simulink model "TRN_V3_2"  (R2022a)
settings: Solver=FixedStepAuto  StartTime=0.0  StopTime=300  FixedStep=0.04  RelTol=1e-3
PreLoadFcn:
  | load('BusStructureTRNsensor.mat');
  | addpath('C:/MAP');
InitFcn:
  | %load TRNDataBusPILS.mat
  | %addpath(genpath(cd))
  | 
  | %load('TPF_WHOLESIM_INPUT_SCENARIOS_AGCAS_N35_10E127_70.mat');
  | 
  | % Add DataBus Path
  | addpath(',,/');
  | addpath('../MAP/');
  | addpath('../MAP/MAP_DB');
  | addpath('../MAP/DVOF');
  | addpath(genpath(cd));
  | load('BusStructureTRN.mat');
undefined symbols (not defined in the file or in its folder): Altitude_INS, Latitude_INS, Longitude_INS, residual, Result_Prev, TimeTag_Prev, TRN, TRNlib
libraries: simulink_extras x21, sharedtransform x2
(part 4 of 4)

== stateflow chart TRN_V3_2/TRN/ModeManagementCSU ==
  state Operation_In_Flight
    state Terrain_Referenced_Navigation [parallel]
      settings: executionOrder=1
      state TrackingCSU
        state ContinuousUpdate [parallel]
          en,du:
          [latINSErrTRN, lonINSErrTRN, altINSErrTRN, Out_TRNOutput.TRNHorUncertainty, ...
          Out_TRNOutput.TRNVerticalUncertainty, Out_TRNDatapump] = TrackingCSU(In_TRNInput,Qmatrix, In_TRNDatapump);
          [continuousValid, Out_TRNOutput.NavigationMode]...
          = CheckValidity( Out_TRNOutput.TRNHorUncertainty, In_TRNInput.INSDataNotValid, In_TRNInput.INS_Alignment_State, ...
          In_TRNInput.GPSDataNotValid);
          [Out_TRNOutput.TRN_Ver_FlightPath_Angle] = Ver_FlightPath_Angle(In_TRNInput);
          settings: executionOrder=1
        state ContinuousValid [parallel]
          en, du:
          [Out_TRNOutput.TRNEstOfINSLatitudeErr, Out_TRNOutput.TRNEstOfINSLongitudeErr, Out_TRNOutput.TRNEstOfINSAltitudeErr, ...
          Out_TRNOutput.AircraftPositionCorrectionValid] ...
          = ValidityCheck(continuousValid, latINSErrTRN, lonINSErrTRN, altINSErrTRN, Out_TRNDatapump.Result_Prev);
          settings: executionOrder=2
      state AcquisitionCSU
        state Batch_On
          state StoreProfile [parallel]
            en, du: [Out_TRNDatapump.MAD, Out_TRNDatapump.profileCnt, posUpdate, Out_TRNDatapump.residual(1)] =...
            AcquisitionCSU(In_TRNInput,In_TRNDatapump);
            settings: executionOrder=1
          state BatchUpdate_Valid [parallel]
            en, du:
            [Out_TRNOutput.TRNEstOfINSLatitudeErr, Out_TRNOutput.TRNEstOfINSLongitudeErr, Out_TRNOutput.TRNEstOfINSAltitudeErr, ...
            Out_TRNDatapump.profileCnt, Out_TRNOutput.NavigationMode, Out_TRNOutput.AircraftPositionCorrectionValid ] = ...
            CorrelationValid(Out_TRNDatapump, In_TRNInput, posUpdate);
            [Out_TRNOutput.TRN_Ver_FlightPath_Angle] = Ver_FlightPath_Angle(In_TRNInput);
            settings: executionOrder=2
        state Batch_Idle
          entry: Out_TRNOutput.TRNEstOfINSLatitudeErr = 0.0;
          Out_TRNOutput.TRNEstOfINSLongitudeErr = 0.0;
          Out_TRNOutput.NavigationMode = true;
          Out_TRNOutput.AircraftPositionCorrectionValid = false;
        (default) -> Batch_On
        Batch_Idle -> Batch_On : after(24, tick)
        Batch_On -> Batch_Idle : after(1, tick)
      (default) -> AcquisitionCSU
      TrackingCSU -> AcquisitionCSU : [In_TRNOutput.NavigationMode == true || ...
          | In_TRNInput.SoftResetRequest == true]
      AcquisitionCSU -> TrackingCSU : [In_TRNOutput.NavigationMode == false]
  state Flight_Idle
    en, du:
    [Out_TRNOutput.TRN_Ver_FlightPath_Angle] = Ver_FlightPath_Angle(In_TRNInput);
    Out_TRNOutput.TRN_valid = true;
    Out_TRNOutput.TRNEstOfINSLatitudeErr = 0.0;
    Out_TRNOutput.TRNEstOfINSLongitudeErr = 0.0;
    Out_TRNOutput.TRNEstOfINSAltitudeErr = 0.0;
    Out_TRNOutput.NavigationMode = false;
    Out_TRNOutput.AircraftPositionCorrectionValid = false;
  state [latINSErrTRN, lonINSErrTRN, altINSErrTRN, hUncertainty, vUncertainty, Out_TRNDatapump] ... [function]
    = TrackingCSU(In_TRNInput,Qmatrix,In_TRNDatapump)
  state [MAD,profileCnt,posUpdate,residual] ... [function]
    = AcquisitionCSU(In_TRNInput,In_TRNDatapump)
  state [TRNEstLatErr,TRNEstLonErr,TRNEstAltErr,profileCnt,NavigationMode,AircraftPositionCorrectionValid] = CorrelationValid(In_TRNDatapump,In_TRNInput,posUpdate) [function]
  state [TRNEstOfINSLatitudeErr,TRNEstOfINSLongitudeErr,TRNEstOfINSAltitudeErr,AircraftPositionCorrectionValid] ... [function]
    = ValidityCheck(continuousValid,latINSErrTRN,lonINSErrTRN,altINSErrTRN,Result_prev)
  state TRN_Ver_FlightPath_Angle = Ver_FlightPath_Angle(In_TRNInput) [function]
  (default) -> Operation_In_Flight
  Operation_In_Flight -> Flight_Idle : [In_TRNInput.WeightOnWheels == true]
  Flight_Idle -> Operation_In_Flight : [In_TRNInput.WeightOnWheels == false]
  data: In_TRNInput function_input Bus: TRNInput size=1 =0; Qmatrix function_input double size=[6 6]; latINSErrTRN function_output; lonINSErrTRN function_output; altINSErrTRN function_output; hUncertainty function_output; vUncertainty function_output; In_TRNDatapump function_input Bus: TRNDatapump size=1; Out_TRNDatapump function_output; In_TRNInput function_input Bus: TRNInput size=1 =0; In_TRNDatapump function_input Bus: TRNDatapump size=1 =0; MAD function_output; profileCnt function_output; posUpdate function_output; residual function_output; In_TRNDatapump function_input Bus: TRNDatapump size=1; TRNEstLatErr function_output; TRNEstLonErr function_output; TRNEstAltErr function_output; In_TRNInput function_input Bus: TRNInput size=1; profileCnt function_output uint32; NavigationMode function_output boolean; AircraftPositionCorrectionValid function_output; posUpdate function_input double size=2; hUncertaintyTRN function_input; INSDataNotValid function_input; valid function_output; navigationMode function_output; INS_Alignment_State function_input; GPSDataNotValid function_input; TRNEstOfINSLatitudeErr function_output; TRNEstOfINSLongitudeErr function_output; TRNEstOfINSAltitudeErr function_output; AircraftPositionCorrectionValid function_output boolean; continuousValid function_input boolean size=1; latINSErrTRN function_input double size=1; lonINSErrTRN function_input double size=1; altINSErrTRN function_input double size=1; Result_prev function_input uint16 size=6; In_TRNInput function_input Bus: TRNInput size=1; TRN_Ver_FlightPath_Angle function_output double; In_TRNInput input Bus: TRNInput; In_TRNOutput input Bus: TRNOutput; In_TRNDatapump input Bus: TRNDatapump; Out_TRNOutput output Bus: TRNOutput; Out_TRNDatapump output Bus: TRNDatapump; Qmatrix input double size=[6 6]; lonINSErrTRN local double; latINSErrTRN local double; altINSErrTRN local double; continuousValid local boolean; posUpdate local
  function [valid, navigationMode] = CheckValidity(hUncertaintyTRN, INSDataNotValid, INS_Alignment_State, GPSDataNotValid):
    | function [valid, navigationMode] = CheckValidity(hUncertaintyTRN, INSDataNotValid, INS_Alignment_State, GPSDataNotValid)
    | 
    | persistent invalidCnt
    | if(isempty(invalidCnt))
    |     invalidCnt = 0;
    | end
    | 
    | 
    | if GPSDataNotValid == true
    |     if(hUncertaintyTRN > (256)) || INS_Alignment_State == false
    |         valid = false;
    |         invalidCnt = invalidCnt + 1;
    |     else
    |         valid = true;
    |         invalidCnt = 0;
    |     end
    | else
    |     if(hUncertaintyTRN > 256)
    |         valid = false;
    |         invalidCnt = invalidCnt + 1;
    |     else
    |         valid = true;
    |         invalidCnt = 0;
    |     end
    | end
    | 
    | if GPSDataNotValid == true
    |     if (invalidCnt > 50) || (INSDataNotValid == true)
    |         navigationMode = true;        % Acq CSU
    |     else
    |         navigationMode = false;       % Track CSU
    |     end
    | else
    |     if (invalidCnt > 50)
    |         navigationMode = true;        % Acq CSU
    |     else
    |         navigationMode = false;       % Track CSU
    |     end
    | end
    | if navigationMode == true
    |     invalidCnt = 0;
    | end
    | end

== matlab function TRN_V3_2/TRN/ModeManagementCSU/AcquisitionCSU/AcquisitionCSU/StoreProfile ==
  data: firstRun input; profileCnt output; batchProfile output; gridSize output; latINS input; lonINS input; altINS input; RALT input; latGPS input; lonGPS input; altGPS input; GPSDataNotValid input; flagINS input; GPSFoM input; batchProfile input; profileCnt input; gridSize input; MAPvalidFlag input
function [profileCnt, batchProfile, gridSize] = StoreProfile(firstRun, latINS, lonINS, altINS, RALT, latGPS, lonGPS, altGPS, GPSDataNotValid, flagINS, GPSFoM, batchProfile, profileCnt, gridSize, MAPvalidFlag)

if (GPSDataNotValid == false) && (GPSFoM <= 2)

    batchProfile((profileCnt*(3+((gridSize + gridSize + 1) * (gridSize + gridSize + 1)))) + 1) = altGPS - RALT;
    batchProfile((profileCnt*(3+((gridSize + gridSize + 1) * (gridSize + gridSize + 1)))) + 2) = latGPS;
    batchProfile((profileCnt*(3+((gridSize + gridSize + 1) * (gridSize + gridSize + 1)))) + 3) = lonGPS;
    
    if firstRun == true
        batchProfile((profileCnt*(3+((gridSize + gridSize + 1) * (gridSize + gridSize + 1)))) + 1) = altINS - RALT;
        batchProfile((profileCnt*(3+((gridSize + gridSize + 1) * (gridSize + gridSize + 1)))) + 2) = latINS;
        batchProfile((profileCnt*(3+((gridSize + gridSize + 1) * (gridSize + gridSize + 1)))) + 3) = lonINS;
    end

else
    batchProfile((profileCnt*(3+((gridSize + gridSize + 1) * (gridSize + gridSize + 1)))) + 1) = altINS - RALT;
    batchProfile((profileCnt*(3+((gridSize + gridSize + 1) * (gridSize + gridSize + 1)))) + 2) = latINS;
    batchProfile((profileCnt*(3+((gridSize + gridSize + 1) * (gridSize + gridSize + 1)))) + 3) = lonINS;

end

if (flagINS == false) && (MAPvalidFlag == true)
    profileCnt = profileCnt + 1;
else
    profileCnt = uint32(0);
end

end

== matlab function TRN_V3_2/TRN/ModeManagementCSU/CorrelationValid/CorrelationValid function ==
  data: posUpdate input; MAD input; profileCnt input; TRNEstOfINSLatitudeErr output; TRNEstOfINSLongitudeErr output; TRNEstOfINSAltitudeErr output; GPSDataNotValid input; profileCnt output; NavigationMode output; AircraftPositionCorrectionValid output
function [TRNEstOfINSLatitudeErr, TRNEstOfINSLongitudeErr, TRNEstOfINSAltitudeErr, profileCnt, NavigationMode, AircraftPositionCorrectionValid] = CorrelationValid(posUpdate, MAD, profileCnt, GPSDataNotValid)

if (MAD < 50 && profileCnt >= 20) || ...
 (GPSDataNotValid == 0 && MAD < 50 && profileCnt >= 5)
    TRNEstOfINSLatitudeErr = -posUpdate(1) * 180/pi;
    TRNEstOfINSLongitudeErr = -posUpdate(2) * 180/pi;
    TRNEstOfINSAltitudeErr = 0.0;
    profileCnt = uint32(0);
    NavigationMode = false;
    AircraftPositionCorrectionValid = true;
else
    TRNEstOfINSLatitudeErr = 0.0;
    TRNEstOfINSLongitudeErr = 0.0;
    TRNEstOfINSAltitudeErr = 0.0;
    NavigationMode = true;
    AircraftPositionCorrectionValid = false;
end
end

== matlab function TRN_V3_2/TRN/ModeManagementCSU/TrackingCSU/TrackingCSU_20230430/Earth_radius ==
  data: M output; N output; Latitude_INS input; psi output
function [M, N, psi] = Earth_radius(Latitude_INS)

    a   = 6378137;          % Earth's equatorial radius
    b   = 6356752.314245;   % Earth's polar radius
    psi = Latitude_INS;     % psi(latitude_INS)
    M   = ((a*b)^2) / ( ( (a*cos(psi))^2 + (b*sin(psi))^2 )^(3/2) );    % radius  of  curvature  in  meridian
    N   = (a^2) / ( ( (a*cos(psi))^2 + (b*sin(psi))^2 )^(1/2) );        % radius  of  curvature  in  prime  vertical

end

== matlab function TRN_V3_2/TRN/ModeManagementCSU/TrackingCSU/TrackingCSU_20230430/INS_Update_1553falt ==
  data: latINS input; latINS output; lonINS input; altINS input; velN input; velE input; velD input; TimeTag input; lonINS output; altINS output; dt input
function [latINS, lonINS, altINS] = INS_Update_1553falt(latINS, lonINS, altINS, velN, velE, velD, TimeTag, dt)

R0 = 6378000;

if TimeTag(5) == 1
    latINS = latINS + (velN * dt) * 1/(R0+altINS);
    lonINS = lonINS + (velE * dt) * 1/(R0+altINS);
    altINS = altINS + (velD * dt) * 1/(R0+altINS);
end

== matlab function TRN_V3_2/TRN/ModeManagementCSU/TrackingCSU/TrackingCSU_20230430/TimeTagCheck ==
  data: TimeTag_Prev input; TimeTag_Prev output; GPStimeValid input; INSTimeTag input; RALTTimeTag input
function TimeTag_Prev   = TimeTagCheck(TimeTag_Prev,GPStimeValid,INSTimeTag,RALTTimeTag)

TimeTag_Prev(4) = 0;
TimeTag_Prev(5) = 0;
TimeTag_Prev(6) = 0;

if TimeTag_Prev(1) == GPStimeValid
    TimeTag_Prev(4) = 1;
end

if TimeTag_Prev(2) == INSTimeTag
    TimeTag_Prev(5) = 1;
end

if TimeTag_Prev(3) == RALTTimeTag
    TimeTag_Prev(6) = 1;
end

TimeTag_Prev(1) = GPStimeValid;
TimeTag_Prev(2) = INSTimeTag;
TimeTag_Prev(3) = RALTTimeTag;
